simulink model "NeuromuscularModelwImpedance"  (R2014b)
settings: Solver=ode15s  StartTime=0.0  StopTime=20  MaxStep=.01  RelTol=1e-4  AbsTol=1e-6
values from neighbouring files (symbols this model uses):
  ankleAngleThr = 2*pi/180    (= 0.0349065850399)    [ControlParams.m]    (also in assignGains.m = Gains(48); saveInitialGuess.m = Gains(40))
  bKneeSwing1 = 0.02    [ControlParams.m]    (also in assignGains.m = Gains(36); saveInitialGuess.m = Gains(28))
  bKneeSwing2 = 0.03    [ControlParams.m]    (also in assignGains.m = Gains(37); saveInitialGuess.m = Gains(29))
  k1AnkleStance1 = 5*180/pi    (= 286.478897565)    [ControlParams.m]    (also in assignGains.m = Gains(38); saveInitialGuess.m = Gains(30))
  k1AnkleStance2 = 5*180/pi    (= 286.478897565)    [ControlParams.m]    (also in assignGains.m = Gains(39); saveInitialGuess.m = Gains(31))
  k1AnkleSwing1 = .5*180/pi    (= 28.6478897565)    [ControlParams.m]    (also in assignGains.m = Gains(40); saveInitialGuess.m = Gains(32))
  k1AnkleSwing2 = 0.75*180/pi    (= 42.9718346348)    [ControlParams.m]    (also in assignGains.m = Gains(41); saveInitialGuess.m = Gains(33))
  k1KneeStance1 = 3.7*180/pi    (= 211.994384198)    [ControlParams.m]    (also in assignGains.m = Gains(42); saveInitialGuess.m = Gains(34))
  k1KneeStance2 = 2.53*180/pi    (= 144.958322168)    [ControlParams.m]    (also in assignGains.m = Gains(43); saveInitialGuess.m = Gains(35))
  k1KneeSwing1 = 0.05*180/pi    (= 2.86478897565)    [ControlParams.m]    (also in assignGains.m = Gains(44); saveInitialGuess.m = Gains(36))
  k1KneeSwing2 = 2.3*180/pi    (= 131.78029288)    [ControlParams.m]    (also in assignGains.m = Gains(45); saveInitialGuess.m = Gains(37))
  k2AnkleStance1 = .5*(180/pi)^3    (= 94045.4744072)    [ControlParams.m]    (also in assignGains.m = Gains(46); saveInitialGuess.m = Gains(38))
  k2KneeStance2 = 7e-4*(180/pi)^3    (= 131.66366417)    [ControlParams.m]    (also in assignGains.m = Gains(47); saveInitialGuess.m = Gains(39))
  LceOffsetTA = 1-0.5*w    [ControlParams.m]
  legLengthClr = .9    (= 0.9)    [ControlParams.m]    (also in assignGains.m = Gains(56); saveInitialGuess.m = Gains(48))
  LongDelay = 0.020    (= 0.02)    [ControlParams.m]
  MidDelay = 0.010    (= 0.01)    [ControlParams.m]
  phiAnkleStance1 = 5*pi/180    (= 0.0872664625997)    [ControlParams.m]    (also in assignGains.m = Gains(49); saveInitialGuess.m = Gains(41))
  phiAnkleStance12 = 2*pi/180    (= 0.0349065850399)    [ControlParams.m]    (also in assignGains.m = Gains(50); saveInitialGuess.m = Gains(42))
  phiAnkleStance2 = 10*pi/180    (= 0.174532925199)    [ControlParams.m]    (also in assignGains.m = Gains(51); saveInitialGuess.m = Gains(43))
  phiHATref = 6*pi/180    (= 0.10471975512)    [ControlParams.m]
  phiKneeStance1 = 8*pi/180    (= 0.13962634016)    [ControlParams.m]    (also in assignGains.m = Gains(52); saveInitialGuess.m = Gains(44))
  phiKneeStance2 = 16*pi/180    (= 0.279252680319)    [ControlParams.m]    (also in assignGains.m = Gains(53); saveInitialGuess.m = Gains(45))
  phiKneeSwing1 = 65*pi/180    (= 1.1344640138)    [ControlParams.m]    (also in assignGains.m = Gains(54); saveInitialGuess.m = Gains(46))
  phiKneeSwing2 = 40*pi/180    (= 0.698131700798)    [ControlParams.m]    (also in assignGains.m = Gains(55); saveInitialGuess.m = Gains(47))
  PreStimGG = 0.05    [ControlParams.m]
  PreStimGLU = 0.01    [ControlParams.m]
  PreStimHAM = 0.01    [ControlParams.m]
  ShortDelay = 0.005    [ControlParams.m]
  simbiconGainD = 5*pi/180    (= 0.0872664625997)    [ControlParams.m]    (also in assignGains.m = Gains(57); saveInitialGuess.m = Gains(49))
  simbiconGainV = 5*pi/180    (= 0.0872664625997)    [ControlParams.m]    (also in assignGains.m = Gains(58); saveInitialGuess.m = Gains(50))
  simbiconLegAngle0 = 85*pi/180    (= 1.4835298642)    [ControlParams.m]    (also in assignGains.m = Gains(59); saveInitialGuess.m = Gains(51))
undefined symbols (not defined in the file or in its folder): DeltaThRef, footCenterToCGDist, footInertia, footMass, g, loptGAS, loptHAMCut, loptTA, lslackGAS, lslackHAMCut, phimaxGASa, phimaxGASk, phirefGASa, phirefGASk, phirefHAMh, rGASa, rGASk, rHAMh, rhoGASa, rhoGASk, rhoHAMh, X, Y, Z
undefined symbols (not defined in the file): RGainGLU, RGainHAM, RhipDGain, RhipPGain, RKglu, RlegAngleFilter, RPosGainGG, RSpeedGainGG
libraries: NeuroMuscularLibrary x67, nesl_utility x16, sm_lib x14, simulink x5, dspswit3 x5, simulink_extras x2
(part 1 of 2)
settings Model: SimulationMode=rapid-accelerator  ParamWorkspaceSource=ReferencedWorkspace  ExtModeTrigDuration=100  TunableVars=LGainGAS,LGainGLU,LGainHAM,LGainKneeOverExt,LGainSOL,LGainSOLTA,LGainTA,LGainVAS,LKglu,LPosGainGG,LSpeedGainGG,LhipDGain,LhipPGain,LkneeExtendGain,LkneeFlexGain,LkneeHoldGain1,LkneeHoldGain2,LkneeStopGain,LlegAngleFilter,RGainGLU,RGainHAM,RKglu,RPosGainGG,RSpeedGainGG,RhipDGain,RhipPGain,RlegAngleFilter,ankleAngleThr,ankleDgain,ankleFilterPID,ankleFilterSEA,anklePgain,bKneeSwing1,bKneeSwing2,groundTheta,groundX,groundZ,impulseTime,impulseValue,k1AnkleStance1,k1AnkleStance2,k1AnkleSwing1,k1AnkleSwing2,k1KneeStance1,k1KneeStance2,k1KneeSwing1,k1KneeSwing2,k2AnkleStance1,k2KneeStance2,kneeDgain,kneeFilterPID,kneeFilterSEA,kneePgain,legLengthClr,phiAnkleStance1,phiAnkleStance12,phiAnkleStance2,phiKneeStance1,phiKneeStance2,phiKneeSwing1,phiKneeSwing2,simbiconGainD,simbiconGainV,simbiconLegAngle0  TunableVarsStorageClass=Auto,Auto,Auto,Auto,Auto,Auto,Auto,Auto,Auto,Auto,Auto,Auto,Auto,Auto,Auto,Auto,Auto,Auto,Auto,Auto,Auto,Auto,Auto,Auto,Auto,Auto,Auto,Auto,Auto,Auto,Auto,Auto,Auto,Auto,Auto,Auto,Auto,Auto,Auto,Auto,Auto,Auto,Auto,Auto,Auto,Auto,Auto,Auto,Auto,Auto,Auto,Auto,Auto,Auto,Auto,Auto,Auto,Auto,Auto,Auto,Auto,Auto,Auto,Auto  TunableVarsTypeQualifier=,,,,,,,,,,,,,,,,,,,,,,,,,,,,,,,,,,,,,,,,,,,,,,,,,,,,,,,,,,,,,,,  Creator=nitisht  LastModifiedBy=Nitish
settings SolverCC: ZeroCrossAlgorithm=Adaptive
settings DataIOCC: SaveFinalState=on  SaveFormat=StructureWithTime  SaveOutput=off  SaveState=on  StateSaveName=tmp_raccel_xout  SignalLoggingName=tmp_raccel_logsout
settings OptimizationCC: InlineParams=on  EfficientMapNaN2IntZero=off  SimCompilerOptimization=On  AccelVerboseBuild=on
settings DebuggingCC: SaveWithDisabledLinksMsg=none  UnderspecifiedInitializationDetection=Classic  MergeDetectMultiDrivingBlocksExec=none  MaxConsecutiveZCsMsg=warning  MaskedZcDiagnostic=none  IgnoredZcDiagnostic=none  StateNameClashWarn=warning
settings HardwareCC: ProdBitPerLong=64  ProdBitPerPointer=64  ProdIntDivRoundTo=Zero  ProdEndianess=LittleEndian  ProdWordSize=64  ProdHWDeviceType=Intel->x86-64  TargetLongLongMode=on  TargetIntDivRoundTo=Zero  TargetEndianess=LittleEndian  TargetHWDeviceType=MATLAB Host  ProdEqTarget=off
settings ModelReferenceCC: UpdateModelReferenceTargets=IfOutOfDate
settings SFSimCC: SFSimEnableDebug=off  SFSimOverflowDetection=off  SFSimEcho=off
settings RTWCC: SystemTargetFile=raccel.tlc  TemplateMakefile=raccel_default_tmf  ProcessScript=raccel_make_rtw_hook  RTWUseSimCustomCode=on
settings CodeAppCC: GenerateComments=off  MaxIdLength=128  MangleLength=10  SimulinkBlockComments=off
settings RaccelTargetCC: ERTMultiwordTypeDef=System defined  ERTMultiwordLength=256  GeneratePreprocessorConditionals=Disable all  ERTFirstTimeCompliant=off  MultiInstanceERTCode=off  EnableShiftOperators=on  ENABLE_SLEXEC_SSBRIDGE=0  RTWCAPIParams=off

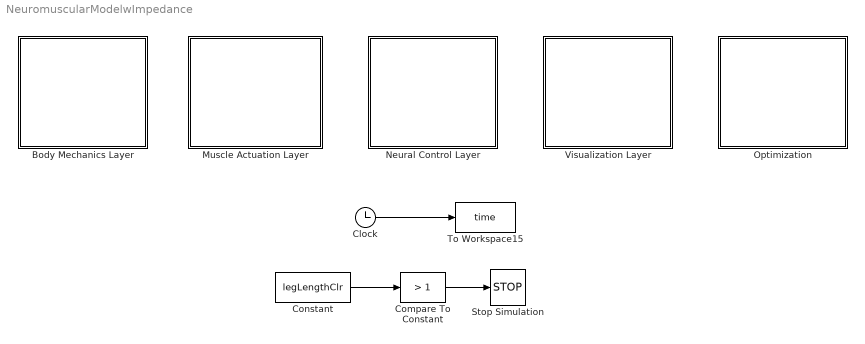
== system NeuromuscularModelwImpedance ==
  Body Mechanics Layer : Subsystem
  Clock : Clock
  Compare To Constant : simulink/Logic and Bit Operations/Compare To Constant  relop=>  const=1  OutDataTypeStr=boolean
  Constant : Constant  Value=legLengthClr
  Muscle Actuation Layer : Subsystem
  Neural Control Layer : Subsystem
  Optimization : Subsystem
  Stop Simulation : Stop
  To Workspace15 : ToWorkspace  VariableName=time  SampleTime=-1
      settings: MaxDataPoints=1
  Visualization Layer : Subsystem
  wires:
  Clock/1 -> To Workspace15/1
  Compare To Constant/1 -> Stop Simulation/1
  Constant/1 -> Compare To Constant/1

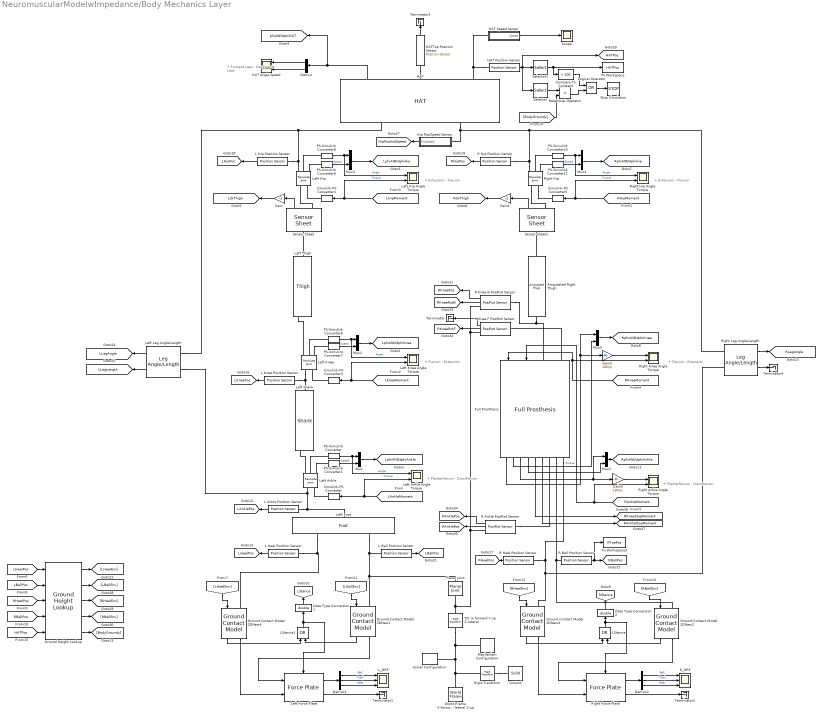
== system NeuromuscularModelwImpedance/Body Mechanics Layer ==
  note: + Flexion
      | -  Extension
  note: + Plantarflexion
      | -  Dorsiflexion
  note: + Extension
      | -  Flexion
  note: + Forward Lean
      | -  Backwards Lean
  note: + Extension
      | -  Flexion
  note: + Flexion
      | -  Extension
  note: + Plantarflexion
      | -  Dorsiflexion
  Amputated Right Thigh : NeuroMuscularLibrary/Amputated Thigh
  Compare To Constant : simulink/Logic and Bit Operations/Compare To Constant  relop=>  const=100  OutDataTypeStr=boolean
  Data Type Conversion1 : DataTypeConversion  OutDataTypeStr=double
  Data Type Conversion2 : DataTypeConversion  OutDataTypeStr=double
  Demux : Demux  Outputs=2
  Demux1 : Demux  Outputs=3
  Demux2 : Demux  Outputs=3
  Full Prosthesis : NeuroMuscularLibrary/Full Prosthesis  SystemSampleTime=-1
  Gain : Gain  Gain=-1
  Gain1 : Gain  Gain=-1
  Gain2 : Gain  Gain=180/pi
  Gain3 : Gain  Gain=180/pi
  Ground : sm_lib/Body Elements/Solid  InertiaType=CalculateFromGeometry  Mass=footMass  MassUnits=kg  CenterOfMass=[-footCenterToCGDist 0 0]  CenterOfMassUnits=m  MomentsOfInertia=[0 0 footInertia]  MomentsOfInertiaUnits=kg*m^2  ProductsOfInertia=[0 0 0]  ProductsOfInertiaUnits=kg*m^2  DensityBased=on  Density=1000  DensityUnits=kg/(m^3)  GraphicType=FromGeometry  MarkerShape=Sphere  MarkerSize=10  MarkerSizeUnits=m  GraphicVisPropType=SimpleVisualProperties  GraphicDiffuseColor=[0.4 0.2 0.0]  GraphicSpecularColor=[0.5 0.5 0.5 1.0]  GraphicAmbientColor=[0.15 0.15 0.15 1.0]  GraphicEmissiveColor=[0.0 0.0 0.0 1.0]  GraphicShininess=75  GraphicOpacity=1.0  GeometryShape=Brick  RectangleSize=[1 1]  RectangleSizeUnits=m  BrickDimensions=[3 1 .01]  BrickDimensionUnits=m  CylinderRadius=1  CylinderRadiusUnits=m  CylinderLength=1  CylinderLengthUnits=m  SphereRadius=1  SphereRadiusUnits=m  EllipsoidRadii=[1 1 1]  EllipsoidRadiiUnits=m  ExtrusionCrossSection=[1 1; -1 1; -1 -1; 1 -1]  ExtrusionCrossSectionUnits=m  ExtrusionLength=1  ExtrusionLengthUnits=m  PolygonNumSides=3  PolygonOuterRadius=1  PolygonOuterRadiusUnits=m  ExtGeomFileType=STL  ExtGeomFileUnits=m  RevolutionCrossSection=[1 1; 1 -1; 2 -1; 2 1]  RevolutionCrossSectionUnits=m  RevolutionExtent=Full  RevolutionAngle=180  RevolutionAngleUnits=deg  BlockFunction=simmechanics.library.body_elements.solid
  Ground Contact Model 2DNew{1..4} (4 alike) : NeuroMuscularLibrary/Ground Contact Model
  Ground Height Lookup : NeuroMuscularLibrary/Ground Height Lookup
  HAT : NeuroMuscularLibrary/HAT
  HAT Position Sensor : NeuroMuscularLibrary/Position Sensor
  HAT Angle Speed : Scope  NumInputPorts=2
      settings: ShowLegends=on  TimeRange=2  YMin=0~-3  YMax=3.25~15  SaveName=ScopeData6
  HAT Speed Sensor : Subsystem
  HATTop Position Sensor : NeuroMuscularLibrary/Position Sensor
  Hip Pos/Speed Sensor : Subsystem
  L Ankle Position Sensor : NeuroMuscularLibrary/Position Sensor
  L Ball Position Sensor : NeuroMuscularLibrary/Position Sensor
  L Heel Position Sensor : NeuroMuscularLibrary/Position Sensor
  L Hip Position Sensor : NeuroMuscularLibrary/Position Sensor
  L Knee Position Sensor : NeuroMuscularLibrary/Position Sensor
  LStance : Logic  Operator=OR  AllPortsSameDT=off  OutDataTypeStr=boolean
  LStance1 : Logic  Operator=OR  AllPortsSameDT=off  OutDataTypeStr=boolean
  L_GRF : Scope  NumInputPorts=3
      settings: ShowLegends=on  TimeRange=0.07974047754022245  YMin=-40~-40~-30  YMax=45~45~130  SaveName=GRF_Heel  SampleTime=0.002
  Left Ankle : sm_lib/Joints/Revolute Joint  SenseConstraintForce=off  SenseConstraintForceX=off  SenseConstraintForceY=off  SenseConstraintForceZ=off  SenseConstraintTorque=off  SenseConstraintTorqueX=off  SenseConstraintTorqueY=off  SenseConstraintTorqueZ=off  SenseTotalForce=off  SenseTotalForceX=off  SenseTotalForceY=off  SenseTotalForceZ=off  SenseTotalTorque=off  SenseTotalTorqueX=off  SenseTotalTorqueY=off  SenseTotalTorqueZ=off  CompositeWrenchDir=FollowerOnBase  CompositeWrenchFrame=BaseFrame  EquilibriumPosition=0  EquilibriumPositionUnits=deg  SpringStiffness=0  SpringStiffnessUnits=N*m/deg  DampingCoefficient=0  DampingCoefficientUnits=N*m/(deg/s)  TorqueActuationMode=InputTorque  MotionActuationMode=ComputedMotion  SensePosition=on  SenseVelocity=on  SenseAcceleration=off  SenseTorqueForce=off  PositionTargetValue=LphiAnkle0  PositionTargetValueUnits=rad  PositionTargetSpecify=on  PositionTargetPriority=High  VelocityTargetValue=0  VelocityTargetValueUnits=rad/s  VelocityTargetSpecify=on  VelocityTargetPriority=Low  BlockFunction=simmechanics.library.joints.revolute_joint
  Left Ankle Angle Torque : Scope  NumInputPorts=2
      settings: ShowLegends=on  TimeRange=3  YMin=-0.6000000000000001~-20  YMax=0.8~140  SaveName=ScopeData4
  Left Foot : NeuroMuscularLibrary/Foot
  Left Force Plate : NeuroMuscularLibrary/Force Plate
  Left Hip : sm_lib/Joints/Revolute Joint  SenseConstraintForce=off  SenseConstraintForceX=off  SenseConstraintForceY=off  SenseConstraintForceZ=off  SenseConstraintTorque=off  SenseConstraintTorqueX=off  SenseConstraintTorqueY=off  SenseConstraintTorqueZ=off  SenseTotalForce=off  SenseTotalForceX=off  SenseTotalForceY=off  SenseTotalForceZ=off  SenseTotalTorque=off  SenseTotalTorqueX=off  SenseTotalTorqueY=off  SenseTotalTorqueZ=off  CompositeWrenchDir=FollowerOnBase  CompositeWrenchFrame=BaseFrame  EquilibriumPosition=0  EquilibriumPositionUnits=deg  SpringStiffness=0  SpringStiffnessUnits=N*m/deg  DampingCoefficient=0  DampingCoefficientUnits=N*m/(deg/s)  TorqueActuationMode=InputTorque  MotionActuationMode=ComputedMotion  SensePosition=on  SenseVelocity=on  SenseAcceleration=off  SenseTorqueForce=off  PositionTargetValue=LphiHip0  PositionTargetValueUnits=rad  PositionTargetSpecify=on  PositionTargetPriority=High  VelocityTargetValue=0  VelocityTargetValueUnits=deg/s  VelocityTargetSpecify=on  VelocityTargetPriority=Low  BlockFunction=simmechanics.library.joints.revolute_joint
  Left Hip Angle Torque : Scope  NumInputPorts=2
      settings: ShowLegends=on  TimeRange=2  YMin=-0.2~-14  YMax=0.8~2  SaveName=ScopeData2
  Left Knee : sm_lib/Joints/Revolute Joint  SenseConstraintForce=off  SenseConstraintForceX=off  SenseConstraintForceY=off  SenseConstraintForceZ=off  SenseConstraintTorque=off  SenseConstraintTorqueX=off  SenseConstraintTorqueY=off  SenseConstraintTorqueZ=off  SenseTotalForce=off  SenseTotalForceX=off  SenseTotalForceY=off  SenseTotalForceZ=off  SenseTotalTorque=off  SenseTotalTorqueX=off  SenseTotalTorqueY=off  SenseTotalTorqueZ=off  CompositeWrenchDir=FollowerOnBase  CompositeWrenchFrame=BaseFrame  EquilibriumPosition=0  EquilibriumPositionUnits=deg  SpringStiffness=0  SpringStiffnessUnits=N*m/deg  DampingCoefficient=0  DampingCoefficientUnits=N*m/(deg/s)  TorqueActuationMode=InputTorque  MotionActuationMode=ComputedMotion  SensePosition=on  SenseVelocity=on  SenseAcceleration=off  SenseTorqueForce=off  PositionTargetValue=LphiKnee0  PositionTargetValueUnits=rad  PositionTargetSpecify=on  PositionTargetPriority=High  VelocityTargetValue=0  VelocityTargetValueUnits=deg/s  VelocityTargetSpecify=on  VelocityTargetPriority=Low  BlockFunction=simmechanics.library.joints.revolute_joint
  Left Knee Angle Torque : Scope  NumInputPorts=2
      settings: ShowLegends=on  TimeRange=2  YMin=-0.1~-100  YMax=1.5~250  SaveName=ScopeData5
  Left Leg Angle/Length : NeuroMuscularLibrary/Leg Angle//Length
  Left Shank : NeuroMuscularLibrary/Shank
  Left Thigh : NeuroMuscularLibrary/Thigh
  Logical Operator : Logic  Operator=OR  AllPortsSameDT=off  OutDataTypeStr=boolean
  Mechanism Configuration : sm_lib/Utilities/Mechanism Configuration  UniformGravity=Constant  GravityVector=[0 0 -g]  GravityUnits=m/s^2  LinearizationDelta=0.001  BlockFunction=simmechanics.library.utilities.mechanism_configuration
  Mux{,1..5} (6 alike) : Mux  Inputs=2
  PS-Simulink Converter{,6,8,10} (4 alike) : nesl_utility/PS-Simulink Converter  PhysicalDomain=network_engine_domain  SubClassName=ps_output  LeftPortType=input  RightPortType=output  PseudoPeriodic=off  Frequencies=[]  Unit=rad  AffineConversion=off
  PS-Simulink Converter{1,7,9,11} (4 alike) : nesl_utility/PS-Simulink Converter  PhysicalDomain=network_engine_domain  SubClassName=ps_output  LeftPortType=input  RightPortType=output  PseudoPeriodic=off  Frequencies=[]  Unit=rad/s  AffineConversion=off
  Planar Joint : sm_lib/Joints/Planar Joint  SenseConstraintForce=off  SenseConstraintForceX=off  SenseConstraintForceY=off  SenseConstraintForceZ=off  SenseConstraintTorque=off  SenseConstraintTorqueX=off  SenseConstraintTorqueY=off  SenseConstraintTorqueZ=off  SenseTotalForce=off  SenseTotalForceX=off  SenseTotalForceY=off  SenseTotalForceZ=off  SenseTotalTorque=off  SenseTotalTorqueX=off  SenseTotalTorqueY=off  SenseTotalTorqueZ=off  CompositeWrenchDir=FollowerOnBase  CompositeWrenchFrame=BaseFrame  PxEquilibriumPosition=0  PxEquilibriumPositionUnits=m  PxSpringStiffness=0  PxSpringStiffnessUnits=N/m  PxDampingCoefficient=0  PxDampingCoefficientUnits=N/(m/s)  PxTorqueActuationMode=NoTorque  PxMotionActuationMode=ComputedMotion  PxSensePosition=off  PxSenseVelocity=off  PxSenseAcceleration=off  PxSenseTorqueForce=off  PxPositionTargetValue=0  PxPositionTargetValueUnits=m  PxPositionTargetSpecify=on  PxPositionTargetPriority=Low  PxVelocityTargetValue=vx0  PxVelocityTargetValueUnits=m/s  PxVelocityTargetSpecify=on  PxVelocityTargetPriority=High  PyEquilibriumPosition=0  PyEquilibriumPositionUnits=m  PySpringStiffness=0  PySpringStiffnessUnits=N/m  PyDampingCoefficient=0  PyDampingCoefficientUnits=N/(m/s)  PyTorqueActuationMode=NoTorque  PyMotionActuationMode=ComputedMotion  PySensePosition=off  PySenseVelocity=off  PySenseAcceleration=off  PySenseTorqueForce=off  PyPositionTargetValue=0  PyPositionTargetValueUnits=m  PyPositionTargetSpecify=on  PyPositionTargetPriority=Low  PyVelocityTargetValue=0  PyVelocityTargetValueUnits=m/s  PyVelocityTargetSpecify=on  PyVelocityTargetPriority=Low  RzEquilibriumPosition=0  RzEquilibriumPositionUnits=deg  RzSpringStiffness=0  RzSpringStiffnessUnits=N*m/deg  RzDampingCoefficient=0  RzDampingCoefficientUnits=N*m/(deg/s)  RzTorqueActuationMode=NoTorque  RzMotionActuationMode=ComputedMotion  RzSensePosition=off  RzSenseVelocity=off  RzSenseAcceleration=off  RzSenseTorqueForce=off  RzPositionTargetValue=0  RzPositionTargetValueUnits=deg  RzPositionTargetSpecify=on  RzPositionTargetPriority=Low  RzVelocityTargetValue=0  RzVelocityTargetValueUnits=deg/s  RzVelocityTargetSpecify=on  RzVelocityTargetPriority=Low  BlockFunction=simmechanics.library.joints.planar_joint
  R Ankle Pos/Rot Sensor : NeuroMuscularLibrary/Pos//Rot Sensor
  R Ball Position Sensor : NeuroMuscularLibrary/Position Sensor
  R Heel Position Sensor : NeuroMuscularLibrary/Position Sensor
  R Hip Position Sensor : NeuroMuscularLibrary/Position Sensor
  R Knee B Pos/Rot Sensor : NeuroMuscularLibrary/Pos//Rot Sensor
  R Knee F Pos/Rot Sensor : NeuroMuscularLibrary/Pos//Rot Sensor
  R_GRF : Scope  NumInputPorts=3
      settings: ShowLegends=on  TimeRange=0.00337774441733929  YMin=50~50~-1  YMax=700~700~1  SaveName=GRF_Heel1  SampleTime=0.002
  Relational Operator : RelationalOperator  Operator=<  OutDataTypeStr=boolean
  Right Ankle Angle Torque : Scope  NumInputPorts=2
      settings: ShowLegends=on  TimeRange=0.35  YMin=-5~-60  YMax=25~60  SaveName=ankleData
  Right Force Plate : NeuroMuscularLibrary/Force Plate
  Right Hip : sm_lib/Joints/Revolute Joint  SenseConstraintForce=off  SenseConstraintForceX=off  SenseConstraintForceY=off  SenseConstraintForceZ=off  SenseConstraintTorque=off  SenseConstraintTorqueX=off  SenseConstraintTorqueY=off  SenseConstraintTorqueZ=off  SenseTotalForce=off  SenseTotalForceX=off  SenseTotalForceY=off  SenseTotalForceZ=off  SenseTotalTorque=off  SenseTotalTorqueX=off  SenseTotalTorqueY=off  SenseTotalTorqueZ=off  CompositeWrenchDir=FollowerOnBase  CompositeWrenchFrame=BaseFrame  EquilibriumPosition=0  EquilibriumPositionUnits=deg  SpringStiffness=0  SpringStiffnessUnits=N*m/deg  DampingCoefficient=0  DampingCoefficientUnits=N*m/(deg/s)  TorqueActuationMode=InputTorque  MotionActuationMode=ComputedMotion  SensePosition=on  SenseVelocity=on  SenseAcceleration=off  SenseTorqueForce=off  PositionTargetValue=RphiHip0  PositionTargetValueUnits=rad  PositionTargetSpecify=on  PositionTargetPriority=High  VelocityTargetValue=0  VelocityTargetValueUnits=deg/s  VelocityTargetSpecify=on  VelocityTargetPriority=Low  BlockFunction=simmechanics.library.joints.revolute_joint
  Right Hip Angle Torque : Scope  NumInputPorts=2
      settings: ShowLegends=on  TimeRange=2  YMin=-0.2~-14  YMax=0.8~2  SaveName=ScopeData12
  Right Knee Angle Torque : Scope  NumInputPorts=2
      settings: ShowLegends=on  TimeRange=1.5  YMin=19~-110  YMax=34~20  SaveName=kneeData
  Right Leg Angle/Length : NeuroMuscularLibrary/Leg Angle//Length
  Rigid Transform : sm_lib/Frames and Transforms/Rigid Transform  TranslationMethod=Cartesian  TranslationLengthUnit=m  TranslationStandardAxis=+X  TranslationStandardOffset=1  TranslationCartesianOffset="[1  0 0]"  TranslationROffset=0  TranslationROffsetUnits=m  TranslationZOffset=0  TranslationZOffsetUnits=m  TranslationThetaOffset=0  TranslationThetaOffsetUnits=deg  RotationMethod=None  RotationAngleUnits=deg  RotationStandardAxis=+Z  RotationAngle=0  RotationArbitraryAxis=[0 0 1]  FollAlignAxisA=+X  BaseAlignAxisA=+Y  FollAlignAxisB=+Y  BaseAlignAxisB=+Z  RotationMatrix=[1 0 0; 0 1 0; 0 0 1]  BlockFunction=simmechanics.library.frames_transforms.rigid_transform
  Scope : Scope
      settings: SaveName=HATSpeed
  Selector : Selector  InputPortWidth=3  Indices=[3]
  Selector1 : Selector  InputPortWidth=3  Indices=[1]
  Sensor Sheet : NeuroMuscularLibrary/Sensor Sheet
  Sensor Sheet1 : NeuroMuscularLibrary/Sensor Sheet
  Simulink-PS Converter{,3..5} (4 alike) : nesl_utility/Simulink-PS Converter  PhysicalDomain=network_engine_domain  SubClassName=ps_input  LeftPortType=input  RightPortType=output  PseudoPeriodic=off  Frequencies=[]  NoiseDistribution=none  NoiseParameters=[]  Unit=N*m  AffineConversion=off  InputFiltering=off  SimscapeFilterOrder=1  InputFilterTimeConstant=0.001  UdotUserProvided=1
  Solver Configuration : nesl_utility/Solver Configuration  PhysicalDomain=network_engine_domain  SubClassName=solver  LeftPortType=input  RightPortType=generic  Accelerate=off  Tones=[]  Harmonics=[]  SimulateNoise=off  Profile=off  UseLocalSampling=off  EnableSwitchedLinearOptims=on  FrequencyDomain=off  UseCCode=off  RelTol=0.001  AbsTol=1e-06  MinStep=1e-09  ToWorkspace=off  DoDC=off  ResidualTolerance=1e-09  UseLocalSolver=off  LocalSolverChoice=NE_BACKWARD_EULER_ADVANCER  LocalSolverSampleTime=0.001  DoFixedCost=off  MaxNonlinIter=3  MaxModeIter=2  LinearAlgebra=Sparse  DelaysMemoryBudget=1024  AutomaticFiltering=on  FilteringTimeConstant=0.001
  Stop Simulation : Stop
  TO: X-forward Y-up Z-lateral : sm_lib/Frames and Transforms/Rigid Transform  TranslationMethod=StandardAxis  TranslationLengthUnit=m  TranslationStandardAxis=+Z  TranslationStandardOffset=hatLeftHipToCenterDistWidth  TranslationCartesianOffset=[0 0 0]  TranslationROffset=0  TranslationROffsetUnits=m  TranslationZOffset=0  TranslationZOffsetUnits=m  TranslationThetaOffset=0  TranslationThetaOffsetUnits=deg  RotationMethod=AlignedAxes  RotationAngleUnits=deg  RotationStandardAxis=+Z  RotationAngle=0  RotationArbitraryAxis=[0 0 1]  FollAlignAxisA=+Z  BaseAlignAxisA=+Y  FollAlignAxisB=+X  BaseAlignAxisB=+X  RotationMatrix=[1 0 0; 0 1 0; 0 0 1]  BlockFunction=simmechanics.library.frames_transforms.rigid_transform
  Terminator{,1..4} (5 alike) : Terminator
  To Workspace : ToWorkspace  VariableName=HATPos  SampleTime=-1
      settings: MaxDataPoints=1
  To Workspace3 : ToWorkspace  VariableName=RToePos  SaveFormat=Structure With Time  SampleTime=-1
  World Frame X-forward Y-lateral Z-up : sm_lib/Frames and Transforms/World Frame  BlockFunction=simmechanics.library.frames_transforms.world_frame
  tag scope: HATPos=global, HipPosAndSpeed=global, LAnklePos=global, LBallPos=global, LHeelPos=global, LHipPos=global, LKneePos=global, LLegAngle=global, LLegLength=global, LStance=global, LdxThigh=global, LphiANDdphiAnkle=global, LphiANDdphiHip=global, LphiANDdphiKnee=global, RAnklePos=global, RAnkleRot=global, RAnkleStopMoment=global, RBallPos=global, RHeelPos=global, RHipPos=global, RKneePos=global, RKneeRotB=global, RKneeRotF=global, RKneeStopMoment=global, RLegAngle=global, RStance=global, RdxThigh=global, RphiANDdphiAnkle=global, RphiANDdphiHip=global, RphiANDdphiKnee=global, phiANDdphiHAT=global
  wires:
  Full Prosthesis/1 -> Mux5/1, Gain2/1
  Gain3/1 -> Right Ankle Angle Torque/1
  Gain2/1 -> Right Knee Angle Torque/1
  Full Prosthesis/2 -> Mux5/2
  Full Prosthesis/4 -> Mux1/2
  Full Prosthesis/3 -> Mux1/1, Gain3/1
  [HATPos] -> Ground Height Lookup/5
  [RBallPos] -> Ground Height Lookup/4
  Ground Height Lookup/5 -> [BodyGroundy]
  Ground Height Lookup/4 -> [RBallEnv]
  Ground Height Lookup/3 -> [RHeelEnv]
  [RHeelPos] -> Ground Height Lookup/3
  Ground Height Lookup/2 -> [LBallEnv]
  [LBallPos] -> Ground Height Lookup/2
  Ground Height Lookup/1 -> [LHeelEnv]
  [LHeelPos] -> Ground Height Lookup/1
  HAT Speed Sensor/1(Speed) -> Scope/1
  [BodyGroundy] -> Relational Operator/2
  HATTop Position Sensor/1 -> Terminator3/1
  Logical Operator/1 -> Stop Simulation/1
  Relational Operator/1 -> Logical Operator/2
  R Knee F Pos/Rot Sensor/1 -> Terminator/1
  Compare To Constant/1 -> Logical Operator/1
  HAT Position Sensor/1 -> Selector1/1, Selector/1, [HATPos]
  R Ankle Pos/Rot Sensor/2 -> [RAnkleRot]
  R Ankle Pos/Rot Sensor/1 -> [RAnklePos]
  R Knee B Pos/Rot Sensor/1 -> [RKneePos]
  R Knee B Pos/Rot Sensor/2 -> [RKneeRotB]
  R Knee F Pos/Rot Sensor/2 -> [RKneeRotF]
  [RBallEnv] -> Ground Contact Model 2DNew2/1
  [RHeelEnv] -> Ground Contact Model 2DNew3/1
  [LBallEnv] -> Ground Contact Model 2DNew1/1
  [LHeelEnv] -> Ground Contact Model 2DNew4/1
  R Heel Position Sensor/1 -> [RHeelPos]
  R Ball Position Sensor/1 -> [RBallPos], To Workspace3/1
  Data Type Conversion2/1 -> [RStance]
  Data Type Conversion1/1 -> [LStance]
  Left Leg Angle/Length/2 -> [LLegLength]
  Left Leg Angle/Length/1 -> [LLegAngle]
  Right Leg Angle/Length/2 -> Terminator4/1
  Right Leg Angle/Length/1 -> [RLegAngle]
  Hip Pos/Speed Sensor/1(PosSpeed) -> [HipPosAndSpeed]
  Selector1/1 -> To Workspace/1, Compare To Constant/1
  Selector/1 -> Relational Operator/1
  PS-Simulink Converter11/1 -> Mux4/2  "Speed"
  PS-Simulink Converter10/1 -> Mux4/1, Right Hip Angle Torque/1  "Angle"
  [RHipMoment] -> Simulink-PS Converter5/1, Right Hip Angle Torque/2  "Torque"
  PS-Simulink Converter8/1 -> Mux3/1, Left Hip Angle Torque/1  "Angle"
  [LHipMoment] -> Simulink-PS Converter4/1, Left Hip Angle Torque/2  "Torque"
  [LAnkleMoment] -> Left Ankle Angle Torque/2, Simulink-PS Converter/1  "Torque"
  [RKneeMoment] -> Full Prosthesis/1, Right Knee Angle Torque/2
  L Ball Position Sensor/1 -> [LBallPos]
  R Hip Position Sensor/1 -> [RHipPos]
  L Hip Position Sensor/1 -> [LHipPos]
  L Knee Position Sensor/1 -> [LKneePos]
  L Heel Position Sensor/1 -> [LHeelPos]
  L Ankle Position Sensor/1 -> [LAnklePos]
  Mux4/1 -> [RphiANDdphiHip]
  [RAnkleMoment] -> Right Ankle Angle Torque/2, Full Prosthesis/2  "Torque"
  Mux1/1 -> [RphiANDdphiAnkle]
  Mux5/1 -> [RphiANDdphiKnee]
  Ground Contact Model 2DNew1/1 -> LStance1/2
  Ground Contact Model 2DNew4/1 -> LStance1/1
  LStance1/1 -> Data Type Conversion1/1, Left Force Plate/Enable
  Ground Contact Model 2DNew2/1 -> LStance/2
  Ground Contact Model 2DNew3/1 -> LStance/1
  Gain1/1 -> [RdxThigh]
  Sensor Sheet1/1 -> Gain1/1
  Gain/1 -> [LdxThigh]
  Mux3/1 -> [LphiANDdphiHip]
  Demux/2 -> HAT Angle Speed/2
  HAT/1 -> Demux/1, [phiANDdphiHAT]
  PS-Simulink Converter9/1 -> Mux3/2  "Speed"
  Sensor Sheet/1 -> Gain/1
  [LKneeMoment] -> Left Knee Angle Torque/2, Simulink-PS Converter3/1
  Mux2/1 -> [LphiANDdphiKnee]
  PS-Simulink Converter1/1 -> Mux/2  "Speed"
  PS-Simulink Converter/1 -> Mux/1, Left Ankle Angle Torque/1  "Angle"
  Demux/1 -> HAT Angle Speed/1
  PS-Simulink Converter7/1 -> Mux2/2  "Speed"
  PS-Simulink Converter6/1 -> Mux2/1, Left Knee Angle Torque/1  "Angle"
  Mux/1 -> [LphiANDdphiAnkle]
  LStance/1 -> Data Type Conversion2/1, Right Force Plate/Enable
  Ground Contact Model 2DNew3/2 -> Right Force Plate/2
  Ground Contact Model 2DNew2/2 -> Right Force Plate/1
  Right Force Plate/2 -> Terminator2/1
  Demux2/3 -> R_GRF/3  "Heel"
  Demux2/2 -> R_GRF/2  "Total"
  Demux2/1 -> R_GRF/1  "Ball"
  Right Force Plate/1 -> Demux2/1
  Ground Contact Model 2DNew4/2 -> Left Force Plate/2
  Ground Contact Model 2DNew1/2 -> Left Force Plate/1
  Left Force Plate/2 -> Terminator1/1
  Demux1/3 -> L_GRF/3  "Heel"
  Demux1/2 -> L_GRF/2  "Total"
  Demux1/1 -> L_GRF/1  "Ball"
  Left Force Plate/1 -> Demux1/1
  Full Prosthesis/6 -> [RAnkleStopMoment]
  Full Prosthesis/5 -> [RKneeStopMoment]
  connections:
  R Ankle Pos/Rot Sensor/LConn1 -- Full Prosthesis/RConn1
  Ground Contact Model 2DNew3/LConn1 -- R Heel Position Sensor/LConn1 -- Full Prosthesis/RConn3 -- Right Leg Angle/Length/LConn2
  HAT Position Sensor/LConn1 -- HAT Speed Sensor/LConn1 -- HAT/RConn2
  R Knee F Pos/Rot Sensor/RConn1 -- TO: X-forward Y-up Z-lateral/LConn1 -- Planar Joint/LConn1 -- R Ankle Pos/Rot Sensor/RConn1 -- R Knee B Pos/Rot Sensor/RConn1
  Left Foot/RConn1 -- L Ankle Position Sensor/LConn1 -- Left Leg Angle/Length/LConn2 -- Left Ankle/LConn1
  HATTop Position Sensor/LConn1 -- HAT/RConn1
  Full Prosthesis/LConn2 -- R Knee F Pos/Rot Sensor/LConn1
  L Ball Position Sensor/LConn1 -- Planar Joint/RConn1 -- Ground Contact Model 2DNew1/LConn1 -- Left Foot/LConn2
  L Heel Position Sensor/LConn1 -- Ground Contact Model 2DNew4/LConn1 -- Left Foot/LConn1
  Left Shank/RConn1 -- L Knee Position Sensor/LConn1 -- Left Knee/LConn1
  Right Hip/RConn1 -- R Hip Position Sensor/LConn1 -- Right Leg Angle/Length/LConn1 -- Hip Pos/Speed Sensor/LConn1 -- HAT/LConn2
  HAT/LConn1 -- Left Leg Angle/Length/LConn1 -- L Hip Position Sensor/LConn1 -- Left Hip/RConn1
  R Ball Position Sensor/LConn1 -- Full Prosthesis/RConn2 -- Ground Contact Model 2DNew2/LConn1
  Amputated Right Thigh/LConn1 -- Full Prosthesis/LConn1 -- R Knee B Pos/Rot Sensor/LConn1
  Right Hip/RConn2 -- PS-Simulink Converter10/LConn1
  Right Hip/RConn3 -- PS-Simulink Converter11/LConn1
  Right Hip/LConn2 -- Simulink-PS Converter5/RConn1
  Right Hip/LConn1 -- Sensor Sheet1/RConn1
  Amputated Right Thigh/RConn1 -- Sensor Sheet1/LConn1
  Left Thigh/RConn1 -- Sensor Sheet/LConn1
  Sensor Sheet/RConn1 -- Left Hip/LConn1
  Rigid Transform/RConn1 -- Ground/RConn1
  Left Hip/RConn3 -- PS-Simulink Converter9/LConn1
  Left Hip/RConn2 -- PS-Simulink Converter8/LConn1
  Simulink-PS Converter4/RConn1 -- Left Hip/LConn2
  Left Knee/RConn3 -- PS-Simulink Converter7/LConn1
  Left Knee/RConn2 -- PS-Simulink Converter6/LConn1
  Simulink-PS Converter3/RConn1 -- Left Knee/LConn2
  Left Ankle/LConn2 -- Simulink-PS Converter/RConn1
  Left Thigh/LConn1 -- Left Knee/RConn1
  Left Ankle/RConn3 -- PS-Simulink Converter1/LConn1
  Left Ankle/RConn2 -- PS-Simulink Converter/LConn1
  Left Ankle/RConn1 -- Left Shank/LConn1
  Solver Configuration/RConn1 -- World Frame X-forward Y-lateral Z-up/RConn1 -- Rigid Transform/LConn1 -- Mechanism Configuration/RConn1 -- TO: X-forward Y-up Z-lateral/RConn1

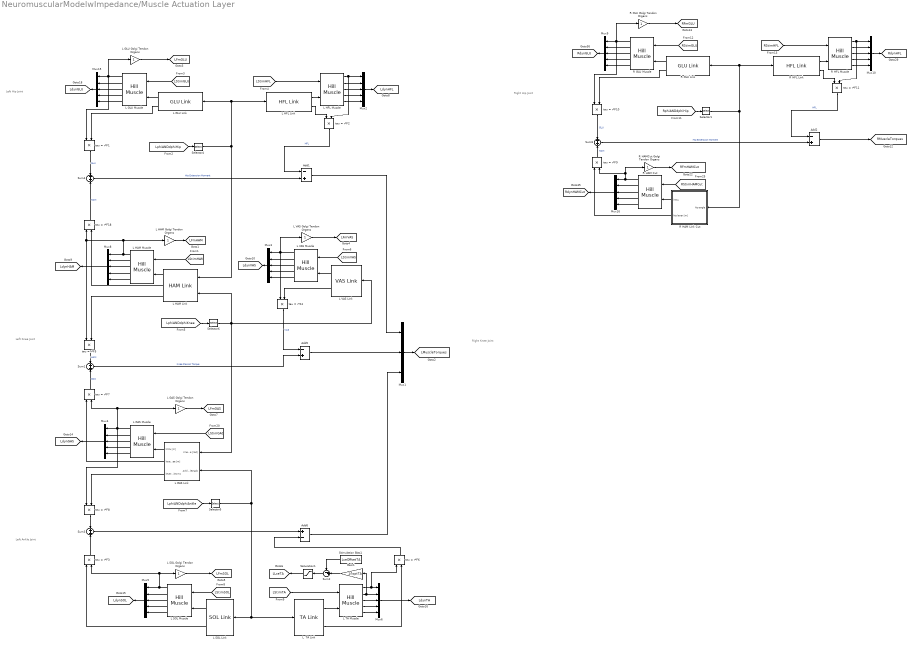
== system NeuromuscularModelwImpedance/Muscle Actuation Layer ==
  note: Left Ankle Joint
  note: Left Knee Joint
  note: Left Hip Joint
  note: Right Knee Joint
  note: Right Hip Joint
  Add1 : Sum  Inputs=-+
  Add2 : Sum  Inputs=-+
  Add5 : Sum  Inputs=-+
  Add6 : Sum  Inputs=+-
  Gain1 : Gain  Gain=1/loptTA
  L  TA Link : NeuroMuscularLibrary/TA Link
  L GAS Golgi Tendon Organs : Gain
  L GAS Link : Subsystem
  L GAS Muscle : NeuroMuscularLibrary/Hill Muscle  Fmax=FmaxGAS  lopt=loptGAS  vmax=vmaxGAS  lslack=lslackGAS
  L GLU Golgi Tendon Organs : Gain
  L GLU Link : NeuroMuscularLibrary/GLU Link
  L GLU Muscle : NeuroMuscularLibrary/Hill Muscle  Fmax=FmaxGLU  lopt=loptGLU  vmax=vmaxGLU  lslack=lslackGLU
  L HAM Golgi Tendon Organs : Gain
  L HAM Link : NeuroMuscularLibrary/HAM Link
  L HAM Muscle : NeuroMuscularLibrary/Hill Muscle  Fmax=FmaxHAM  lopt=loptHAM  vmax=vmaxHAM  lslack=lslackHAM
  L HFL Link : NeuroMuscularLibrary/HFL Link
  L HFL Muscle : NeuroMuscularLibrary/Hill Muscle  Fmax=FmaxHFL  lopt=loptHFL  vmax=vmaxHFL  lslack=lslackHFL
  L SOL Golgi Tendon Organs : Gain
  L SOL Link : NeuroMuscularLibrary/SOL Link
  L SOL Muscle : NeuroMuscularLibrary/Hill Muscle  Fmax=FmaxSOL  lopt=loptSOL  vmax=vmaxSOL  lslack=lslackSOL
  L TA Muscle : NeuroMuscularLibrary/Hill Muscle  Fmax=FmaxTA  lopt=loptTA  vmax=vmaxTA  lslack=lslackTA
  L VAS Golgi Tendon Organs : Gain
  L VAS Link : NeuroMuscularLibrary/VAS Link
  L VAS Muscle : NeuroMuscularLibrary/Hill Muscle  Fmax=FmaxVAS  lopt=loptVAS  vmax=vmaxVAS  lslack=lslackVAS
  Mux1 : Mux  Inputs=3
  Mux{2..6,8..10,15..16} (10 alike) : Mux  Inputs=5
  R GLU Golgi Tendon Organs : Gain
  R GLU Link : NeuroMuscularLibrary/GLU Link
  R GLU Muscle : NeuroMuscularLibrary/Hill Muscle  Fmax=FmaxGLU  lopt=loptGLU  vmax=vmaxGLU  lslack=lslackGLU
  R HAM Cut : NeuroMuscularLibrary/Hill Muscle  Fmax=FmaxHAMCut  lopt=loptHAMCut  vmax=vmaxHAM  lslack=lslackHAMCut
  R HAM Link Cut : Subsystem
  R HAMCut Golgi Tendon Organs : Gain
  R HFL Link : NeuroMuscularLibrary/HFL Link
  R HFL Muscle : NeuroMuscularLibrary/Hill Muscle  Fmax=FmaxHFL  lopt=loptHFL  vmax=vmaxHFL  lslack=lslackHFL
  Saturation1 : Saturate  UpperLimit=inf  LowerLimit=0
  Selector{1,4..6} (4 alike) : Selector  InputPortWidth=2
  Stimulation Bias1 : Constant  Value=LceOffsetTA
  Sum{1,3..4,8} (4 alike) : Sum  Inputs=+|+
  Sum2 : Sum  Inputs=-+|
  tau = r*F{1..11,18} (12 alike) : Product
  tag scope: LFmGAS=global, LFmGLU=global, LFmHAM=global, LFmSOL=global, LFmVAS=global, LLceTA=global, LMuscleTorques=global, LdynGAS=global, LdynGLU=global, LdynHAM=global, LdynHFL=global, LdynSOL=global, LdynTA=global, LdynVAS=global, RFmGLU=global, RFmHAMCut=global, RMuscleTorques=global, RdynGLU=global, RdynHAMCut=global, RdynHFL=global
  wires:
  R HAMCut Golgi Tendon Organs/1 -> [RFmHAMCut]
  Mux16/1 -> [RdynHAMCut]
  R HAM Link Cut/2(hip lever [m]) -> tau = r*F9/1
  R HAM Link Cut/1(lmtu) -> R HAM Cut/2
  [RStimHAMCut] -> R HAM Cut/1
  R HAM Cut/1 -> R HAMCut Golgi Tendon Organs/1, tau = r*F9/2, Mux16/1
  R HAM Cut/2 -> Mux16/2
  R HAM Cut/4 -> Mux16/4
  R HAM Cut/3 -> Mux16/3
  R HAM Cut/5 -> Mux16/5
  Selector1/1 -> R HFL Link/1, R GLU Link/1, R HAM Link Cut/1(hip angle)
  Mux1/1 -> [LMuscleTorques]
  Mux15/1 -> [LdynGLU]
  L TA Muscle/2 -> Mux6/2, Gain1/1
  tau = r*F4/1 -> Add5/1  "VAS"
  tau = r*F5/1 -> Sum1/1  "HAM"
  tau = r*F7/1 -> Sum1/2  "GAS"
  Sum4/1 -> Add1/2  "Hip Extension Moment"
  L HAM Muscle/1 -> Mux8/1, L HAM Golgi Tendon Organs/1, tau = r*F18/1, tau = r*F5/1
  tau = r*F2/1 -> Add1/1  "HFL"
  tau = r*F1/1 -> Sum4/1  "GLU"
  tau = r*F18/1 -> Sum4/2  "HAM"
  L GAS Golgi Tendon Organs/1 -> [LFmGAS]
  L GAS Muscle/1 -> tau = r*F8/1, L GAS Golgi Tendon Organs/1, tau = r*F7/2, Mux4/1
  tau = r*F8/1 -> Sum3/1
  L GAS Link/3(leverAnkle [m]) -> tau = r*F8/2
  Sum3/1 -> Add6/1
  tau = r*F3/1 -> Sum3/2
  [LStimGAS] -> L GAS Muscle/1
  L GAS Link/2(leverKnee [m]) -> tau = r*F7/1
  L GAS Muscle/4 -> Mux4/4
  L GAS Muscle/3 -> Mux4/3
  L GAS Muscle/2 -> Mux4/2
  Mux4/1 -> [LdynGAS]
  L GAS Muscle/5 -> Mux4/5
  Selector6/1 -> L GAS Link/1(Knee Angle [rad]), L VAS Link/1, L HAM Link/2
  L GAS Link/1(lmtu [m]) -> L GAS Muscle/2
  tau = r*F6/1 -> Add6/2
  L  TA Link/2 -> tau = r*F6/2
  Stimulation Bias1/1 -> Sum2/1
  Gain1/1 -> Sum2/2
  [LStimTA] -> L TA Muscle/1
  Saturation1/1 -> [LLceTA]
  Sum2/1 -> Saturation1/1
  L TA Muscle/3 -> Mux6/3
  L TA Muscle/4 -> Mux6/4
  Mux6/1 -> [LdynTA]
  L TA Muscle/5 -> Mux6/5
  L TA Muscle/1 -> Mux6/1, tau = r*F6/1
  L  TA Link/1 -> L TA Muscle/2
  Add6/1 -> Mux1/3
  [LphiANDdphiAnkle] -> Selector5/1
  Selector5/1 -> L GAS Link/2(Ankle Angle[rad]), L SOL Link/1, L  TA Link/1
  [LStimSOL] -> L SOL Muscle/1
  L SOL Golgi Tendon Organs/1 -> [LFmSOL]
  L SOL Link/1 -> L SOL Muscle/2
  L SOL Link/2 -> tau = r*F3/1
  L SOL Muscle/4 -> Mux5/4
  L SOL Muscle/3 -> Mux5/3
  L SOL Muscle/2 -> Mux5/2
  Mux5/1 -> [LdynSOL]
  L SOL Muscle/5 -> Mux5/5
  L SOL Muscle/1 -> Mux5/1, tau = r*F3/2, L SOL Golgi Tendon Organs/1
  [LphiANDdphiKnee] -> Selector6/1
  [LStimVAS] -> L VAS Muscle/1
  Sum1/1 -> Add5/2  "Knee Flexion Torque"
  L HAM Link/3 -> tau = r*F5/2
  L VAS Link/2 -> tau = r*F4/2
  L VAS Golgi Tendon Organs/1 -> [LFmVAS]
  L VAS Muscle/1 -> tau = r*F4/1, Mux3/1, L VAS Golgi Tendon Organs/1
  L VAS Muscle/4 -> Mux3/4
  L VAS Muscle/3 -> Mux3/3
  L VAS Muscle/2 -> Mux3/2
  Mux3/1 -> [LdynVAS]
  L VAS Muscle/5 -> Mux3/5
  L VAS Link/1 -> L VAS Muscle/2
  Add5/1 -> Mux1/2
  [LStimHAM] -> L HAM Muscle/1
  L HAM Golgi Tendon Organs/1 -> [LFmHAM]
  L HAM Muscle/2 -> Mux8/2
  L HFL Muscle/1 -> tau = r*F2/2, Mux2/1
  L HFL Link/2 -> tau = r*F2/1
  L HFL Muscle/3 -> Mux2/3
  L HFL Muscle/4 -> Mux2/4
  Mux2/1 -> [LdynHFL]
  L HFL Muscle/5 -> Mux2/5
  L HFL Muscle/2 -> Mux2/2
  [LStimHFL] -> L HFL Muscle/1
  L HFL Link/1 -> L HFL Muscle/2
  L GLU Golgi Tendon Organs/1 -> [LFmGLU]
  L GLU Muscle/1 -> tau = r*F1/1, L GLU Golgi Tendon Organs/1, Mux15/1
  L GLU Link/2 -> tau = r*F1/2
  L GLU Muscle/4 -> Mux15/4
  L GLU Muscle/3 -> Mux15/3
  L GLU Muscle/2 -> Mux15/2
  L GLU Muscle/5 -> Mux15/5
  [LStimGLU] -> L GLU Muscle/1
  L GLU Link/1 -> L GLU Muscle/2
  Add1/1 -> Mux1/1
  Selector4/1 -> L HFL Link/1, L GLU Link/1, L HAM Link/1
  [LphiANDdphiHip] -> Selector4/1
  L HAM Muscle/4 -> Mux8/4
  L HAM Muscle/3 -> Mux8/3
  Mux8/1 -> [LdynHAM]
  L HAM Muscle/5 -> Mux8/5
  L HAM Link/2 -> tau = r*F18/2
  L HAM Link/1 -> L HAM Muscle/2
  Add2/1 -> [RMuscleTorques]
  Mux9/1 -> [RdynGLU]
  Sum8/1 -> Add2/2  "Hip Extension Moment"
  tau = r*F11/1 -> Add2/1  "HFL"
  tau = r*F10/1 -> Sum8/1  "GLU"
  tau = r*F9/1 -> Sum8/2  "HAM"
  R HFL Muscle/1 -> tau = r*F11/2, Mux10/1
  R HFL Link/2 -> tau = r*F11/1
  R HFL Muscle/3 -> Mux10/3
  R HFL Muscle/4 -> Mux10/4
  Mux10/1 -> [RdynHFL]
  R HFL Muscle/5 -> Mux10/5
  R HFL Muscle/2 -> Mux10/2
  [RStimHFL] -> R HFL Muscle/1
  R HFL Link/1 -> R HFL Muscle/2
  R GLU Golgi Tendon Organs/1 -> [RFmGLU]
  R GLU Muscle/1 -> tau = r*F10/1, R GLU Golgi Tendon Organs/1, Mux9/1
  R GLU Link/2 -> tau = r*F10/2
  R GLU Muscle/4 -> Mux9/4
  R GLU Muscle/3 -> Mux9/3
  R GLU Muscle/2 -> Mux9/2
  R GLU Muscle/5 -> Mux9/5
  [RStimGLU] -> R GLU Muscle/1
  R GLU Link/1 -> R GLU Muscle/2
  [RphiANDdphiHip] -> Selector1/1

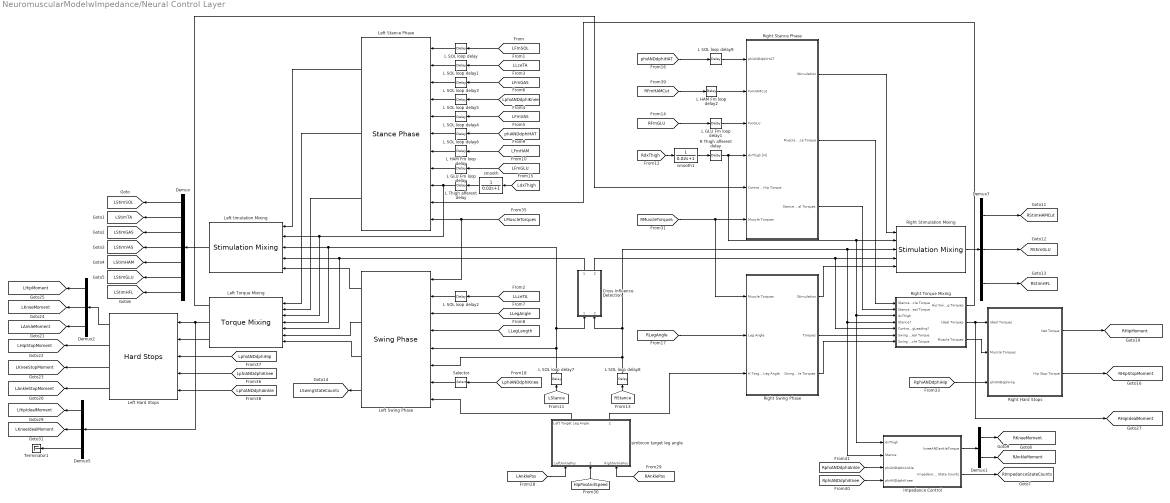
== system NeuromuscularModelwImpedance/Neural Control Layer ==
  Cross Influence Detection : Subsystem
  Demux : Demux  Outputs=7
  Demux1 : Demux  Outputs=2
  Demux2 : Demux  Outputs=3
  Demux5 : Demux  Outputs=3
  Demux7 : Demux  Outputs=3
  Impedance Control : Subsystem
  L GLU Fm loop delay : TransportDelay  DelayTime=ShortDelay
  L GLU Fm loop delay1 : TransportDelay  DelayTime=ShortDelay
  L HAM Fm loop delay : TransportDelay  DelayTime=ShortDelay
  L HAM Fm loop delay2 : TransportDelay  DelayTime=ShortDelay  BufferSize=2048
  L SOL loop delay{,1..3} (4 alike) : TransportDelay  DelayTime=LongDelay
  L SOL loop delay{4..5,7..8} (4 alike) : TransportDelay  DelayTime=MidDelay
  L SOL loop delay6 : TransportDelay  DelayTime=ShortDelay
  L SOL loop delay9 : TransportDelay  DelayTime=ShortDelay
  L Thigh afferent delay : TransportDelay  DelayTime=ShortDelay
  Left Hard Stops : NeuroMuscularLibrary/Hard Stops
  Left Stance Phase : NeuroMuscularLibrary/Stance Phase  GainHAM=LGainHAM  GainGLU=LGainGLU  GainSOL=LGainSOL  GainSOLTA=LGainSOLTA  GainTA=LGainTA  GainGAS=LGainGAS  GainVAS=LGainVAS  GainKneeOverExt=LGainKneeOverExt  PosGainGG=LPosGainGG  SpeedGainGG=LSpeedGainGG  Kglu=LKglu
  Left Swing Phase : NeuroMuscularLibrary/Swing Phase  GainTA=LGainTA  hipPGain=LhipPGain  hipDGain=LhipDGain  legAngleFilter=LlegAngleFilter  kneeFlexGain=LkneeFlexGain  kneeHoldGain1=LkneeHoldGain1  kneeHoldGain2=LkneeHoldGain2  kneeStopGain=LkneeStopGain  kneeExtendGain=LkneeExtendGain  legLengthClr=legLengthClr
  Left Torque Mixing : NeuroMuscularLibrary/Torque Mixing
  Left timulation Mixing : NeuroMuscularLibrary/Stimulation Mixing
  R Thigh afferent delay : TransportDelay  DelayTime=ShortDelay
  Right Hard Stops : Subsystem
  Right Stance Phase : Subsystem  mask{GainHAM=RGainHAM, GainGLU=RGainGLU, PosGainGG=RPosGainGG, SpeedGainGG=RSpeedGainGG, Kglu=RKglu}
  Right Stimulation Mixing : NeuroMuscularLibrary/Stimulation Mixing
  Right Swing Phase : Subsystem  mask{hipPGain=RhipPGain, hipDGain=RhipDGain, legAngleFilter=RlegAngleFilter}
  Right Torque Mixing : Subsystem
  Selector : Selector  InputPortWidth=2  Indices=2
  Terminator1 : Terminator
  simbicon target leg angle : Subsystem
  smooth : TransferFcn  Denominator=[0.02 1]
  smooth1 : TransferFcn  Denominator=[0.02 1]
  tag scope: LAnkleMoment=global, LAnkleStopMoment=global, LHipIdealMoment=global, LHipMoment=global, LHipStopMoment=global, LKneeIdealMoment=global, LKneeMoment=global, LKneeStopMoment=global, LStimGAS=global, LStimGLU=global, LStimHAM=global, LStimHFL=global, LStimSOL=global, LStimTA=global, LStimVAS=global, LSwingStateCounts=global, RAnkleMoment=global, RHipIdealMoment=global, RHipMoment=global, RHipStopMoment=global, RImpedanceStateCounts=global, RKneeMoment=global, RStimGLU=global, RStimHAMCut=global, RStimHFL=global
  wires:
  [RFmHAMCut] -> L HAM Fm loop delay2/1
  L GLU Fm loop delay1/1 -> Right Stance Phase/3(FmGLU)
  Demux5/3 -> Terminator1/1
  Demux5/2 -> [LKneeIdealMoment]
  Demux5/1 -> [LHipIdealMoment]
  Left Swing Phase/3 -> Left Torque Mixing/7
  Left Swing Phase/2 -> Left Torque Mixing/6
  Left Stance Phase/3 -> Left Torque Mixing/2
  Left Torque Mixing/1 -> Right Stance Phase/5(Contra Swing Hip Torque)
  Left Torque Mixing/3 -> Left Hard Stops/2
  Left Torque Mixing/2 -> Left Hard Stops/1, Demux5/1
  [LphiANDdphiAnkle] -> Left Hard Stops/5
  Right Torque Mixing/1(Hip Swing Torques) -> Left Stance Phase/10
  Right Torque Mixing/3(Muscle Torques) -> Right Hard Stops/2(Muscle Torques)
  Right Stance Phase/2(Muscle Stance Torque) -> Right Torque Mixing/1(Stance Muscle Torque)
  Right Stance Phase/3(Stance Ideal Torques) -> Right Torque Mixing/2(Stance Ideal Torque)
  Right Swing Phase/2(Torques) -> Right Torque Mixing/6(Swing Ideal Torque)
  Right Swing Phase/3(Swing Muscle Torques) -> Right Torque Mixing/7(Swing Muscle Torque)
  Right Torque Mixing/2(Ideal Torques) -> [RHipIdealMoment], Right Hard Stops/1(Ideal Torques)
  [RMuscleTorques] -> Right Swing Phase/1(Muscle Torques), Right Stance Phase/6(Muscle Torques)
  Demux2/2 -> [LKneeMoment]
  Left Stance Phase/2 -> Left Torque Mixing/1
  Left Hard Stops/4 -> [LAnkleStopMoment]
  Left Hard Stops/3 -> [LKneeStopMoment]
  Left Hard Stops/2 -> [LHipStopMoment]
  [LphiANDdphiHip] -> Left Hard Stops/3
  [LphiANDdphiKnee] -> Left Hard Stops/4
  Left Hard Stops/1 -> Demux2/1
  Demux2/3 -> [LAnkleMoment]
  Demux2/1 -> [LHipMoment]
  [LMuscleTorques] -> Left Stance Phase/11, Left Swing Phase/1
  Right Hard Stops/2(Hip Stop Torque) -> [RHipStopMoment]
  [RphiANDdphiHip] -> Right Hard Stops/3(phiANDdphiHip)
  Left Swing Phase/4 -> [LSwingStateCounts]
  simbicon target leg angle/1(Left Target Leg Angle) -> Left Swing Phase/8
  simbicon target leg angle/2(Right Target Leg Angle) -> Right Swing Phase/3(H Target Leg Angle)
  [HipPosAndSpeed] -> simbicon target leg angle/2(HIPposAndSpeed)
  Left Swing Phase/1 -> Left timulation Mixing/5
  Selector/1 -> Left Swing Phase/7
  [LphiANDdphiKnee] -> Selector/1
  Right Swing Phase/1(Stimulation) -> Right Stimulation Mixing/5
  [RAnklePos] -> simbicon target leg angle/3(RightAnklePos)
  [LAnklePos] -> simbicon target leg angle/1(LeftAnklePos)
  [RLegAngle] -> Right Swing Phase/2(Leg Angle)
  [LLegLength] -> Left Swing Phase/4
  [LLegAngle] -> Left Swing Phase/3
  Right Hard Stops/1(Net Torque) -> [RHipMoment]
  Cross Influence Detection/1(RightLeading) -> Left timulation Mixing/4, Left Torque Mixing/5
  Left Stance Phase/1 -> Left timulation Mixing/1
  Left timulation Mixing/1 -> Demux/1
  Cross Influence Detection/2(LeftLeading) -> Right Stimulation Mixing/4, Right Torque Mixing/5(ContraLegLeading?)
  Right Stance Phase/1(Stimulation) -> Right Stimulation Mixing/1
  L SOL loop delay2/1 -> Left Swing Phase/2
  L GLU Fm loop delay/1 -> Left Stance Phase/8
  L HAM Fm loop delay/1 -> Left Stance Phase/7
  L Thigh afferent delay/1 -> Left Stance Phase/9, Left timulation Mixing/2, Left Torque Mixing/3
  [RStance] -> L SOL loop delay8/1
  [LStance] -> L SOL loop delay7/1
  L SOL loop delay9/1 -> Right Stance Phase/1(phiANDdphiHAT)
  [phiANDdphiHAT] -> L SOL loop delay9/1
  [RFmGLU] -> L GLU Fm loop delay1/1
  L SOL loop delay7/1 -> Left Swing Phase/5, Cross Influence Detection/1(LStance), Left timulation Mixing/3, Left Torque Mixing/4
  [LFmGLU] -> L GLU Fm loop delay/1
  [LFmHAM] -> L HAM Fm loop delay/1
  smooth1/1 -> R Thigh afferent delay/1
  [RdxThigh] -> smooth1/1
  smooth/1 -> L Thigh afferent delay/1
  [LdxThigh] -> smooth/1
  Demux/7 -> [LStimHFL]
  Demux/6 -> [LStimGLU]
  Demux/5 -> [LStimHAM]
  L SOL loop delay6/1 -> Left Stance Phase/6
  [phiANDdphiHAT] -> L SOL loop delay6/1
  Demux/4 -> [LStimVAS]
  [LphiANDdphiKnee] -> L SOL loop delay5/1
  L SOL loop delay5/1 -> Left Stance Phase/4
  [LFmVAS] -> L SOL loop delay4/1
  L SOL loop delay4/1 -> Left Stance Phase/5
  [LLceTA] -> L SOL loop delay2/1
  L SOL loop delay3/1 -> Left Stance Phase/3
  [LFmGAS] -> L SOL loop delay3/1
  Demux/3 -> [LStimGAS]
  Demux/2 -> [LStimTA]
  Demux/1 -> [LStimSOL]
  L SOL loop delay1/1 -> Left Stance Phase/2
  [LLceTA] -> L SOL loop delay1/1
  L SOL loop delay/1 -> Left Stance Phase/1
  [LFmSOL] -> L SOL loop delay/1
  R Thigh afferent delay/1 -> Right Stimulation Mixing/2, Right Torque Mixing/3(dxThigh), Impedance Control/1(dxThigh), Right Stance Phase/4(dxThigh [N])
  [RphiANDdphiKnee] -> Impedance Control/4(phiANDdphiKnee)
  [RphiANDdphiAnkle] -> Impedance Control/3(phiANDdphiAnkle)
  L SOL loop delay8/1 -> Left Swing Phase/6, Cross Influence Detection/2(RStance), Right Stimulation Mixing/3, Impedance Control/2(Stance), Right Torque Mixing/4(Stance?)
  Impedance Control/1(kneeANDankleTorque) -> Demux1/1
  Demux1/1 -> [RKneeMoment]
  Demux1/2 -> [RAnkleMoment]
  Impedance Control/2(Impedance State Counts) -> [RImpedanceStateCounts]
  Demux7/1 -> [RStimHAMCut]
  Demux7/3 -> [RStimHFL]
  Demux7/2 -> [RStimGLU]
  Right Stimulation Mixing/1 -> Demux7/1
  L HAM Fm loop delay2/1 -> Right Stance Phase/2(FmHAMCut)
